simulink model "FuzzyLogicImplementation"  (R2023a)
settings: Solver=VariableStepAuto  StartTime=0.0  StopTime=10.0  RelTol=1e-3
libraries: fuzblock x1
settings Model: Creator=Chetan Varma  LastModifiedBy=Chetan Varma

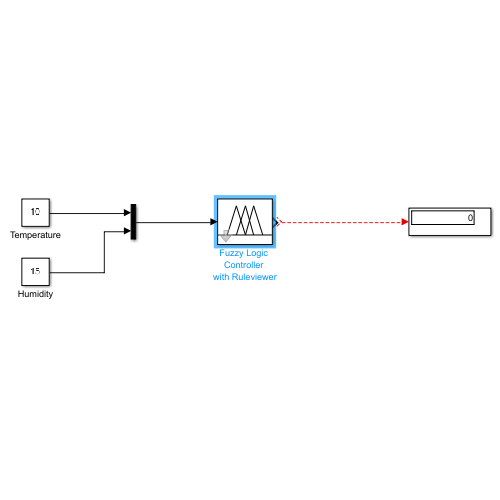
[thumbnail: Simulink's stored preview of the top-level diagram]
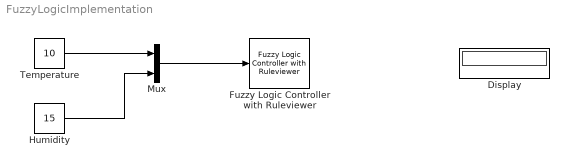
== system FuzzyLogicImplementation ==
  Display : Display
  Fuzzy Logic Controller with Ruleviewer : fuzblock/Fuzzy Logic  Controller  with Ruleviewer  fismatrix=Cooling_System  Ts=2
  Humidity : Constant  Value=15
  Mux : Mux  Inputs=2
  Temperature : Constant  Value=10
  wires:
  Temperature/1 -> Mux/1
  Humidity/1 -> Mux/2
  Mux/1 -> Fuzzy Logic Controller with Ruleviewer/1
  ? -> Display/1
